simulink model "main_model"  (R2018b)
settings: Solver=VariableStepAuto  StartTime=0.0  StopTime=1  RelTol=1e-10
values from neighbouring files (symbols this model uses):
  ba = Jeq*omega_pos*n;       disp("    ba = " + ba)    [control_design.m]
  beq = bm + bl/r^2    (= 1.5e-05)    [data.m]
  Cts = 1.091    [data.m]
  Jeq = Jm + Jl/r^2    (= 5.65099476805e-06)    [data.m]
  ksa = Jeq*omega_pos^2*n;    disp("    ksa = " + ksa)    [control_design.m]
  ksia = Jeq*omega_pos^3;     disp("    ksia = " + ksia)    [control_design.m]
  lambda_rm = 0.01546    [data.m]
  Ld = 6.6e-3    (= 0.0066)    [data.m]
  Lls = 0.8e-3    (= 0.0008)    [data.m]
  Lq = 5.8e-3    (= 0.0058)    [data.m]
  Pp = 3    [data.m]
  r = 314.3008    [data.m]
  R0p = Lls*p;    disp("    R0p = " + R0p)    [control_design.m]    (also in torque_modulator.m = Lls*p;    disp("R0p = " + R0p))
  Rdp = Ld*p;     disp("    Rdp = " + Rdp)    [control_design.m]    (also in torque_modulator.m = Ld*p;     disp("Rdp = " + Rdp))
  Rqp = Lq*p;     disp("    Rqp = " + Rqp)    [control_design.m]    (also in torque_modulator.m = Lq*p;     disp("Rqp = " + Rqp))
  Rs = 1.02    [data.m]
  Rts_amb = 55    [data.m]
  Tamb_max = 40    [data.m]
undefined symbols (not defined in the file or in its folder): lamb
settings Model: Creator=Acer  LastModifiedBy=Acer

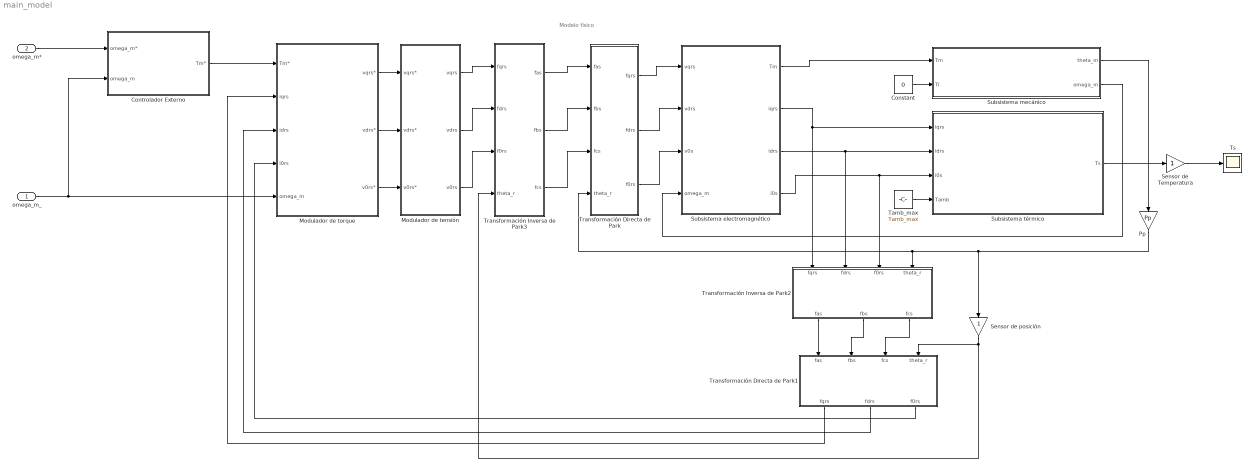
== system main_model ==
  note: Modelo físico
  omega_m_ : Inport
  omega_m* : Inport  Port=2
  " Sensor de posición" : Gain
  Constant : Constant  Value=0
  Controlador Externo : Subsystem
  Modulador de tensión : Subsystem
  Modulador de torque : Subsystem
  Pp : Gain  Gain=Pp
  Sensor de Temperatura : Gain
  Subsistema electromagnético : Subsystem
  Subsistema mecánico : Subsystem
  Subsistema térmico : Subsystem
  Tamb_max : Constant  Value=Tamb_max
  Transformación Directa de Park : MATLAB Function  TreatAsAtomicUnit=on
  Transformación Directa de Park1 : MATLAB Function  TreatAsAtomicUnit=on
  Transformación Inversa de Park2 : MATLAB Function  TreatAsAtomicUnit=on
  Transformación Inversa de Park3 : MATLAB Function  TreatAsAtomicUnit=on
  Ts : Scope
  wires:
  Subsistema mecánico/1(theta_m) -> Pp/1
  Subsistema mecánico/2(omega_m) -> Subsistema electromagnético/4(omega_m)
  Subsistema electromagnético/2(iqrs) -> Transformación Inversa de Park2/1(fqrs), Subsistema térmico/1(iqrs)
  Subsistema electromagnético/1(Tm) -> Subsistema mecánico/1(Tm)
  Subsistema electromagnético/4(i0s) -> Subsistema térmico/3(i0s), Transformación Inversa de Park2/3(f0rs)
  Subsistema térmico/1(Ts) -> Sensor de Temperatura/1
  Tamb_max/1 -> Subsistema térmico/4(Tamb)
  Pp/1 -> " Sensor de posición"/1, Transformación Directa de Park/4(theta_r), Transformación Inversa de Park2/4(theta_r)
  Subsistema electromagnético/3(idrs) -> Subsistema térmico/2(idrs), Transformación Inversa de Park2/2(fdrs)
  Modulador de tensión/1(vqrs) -> Transformación Inversa de Park3/1(fqrs)
  Modulador de tensión/2(vdrs) -> Transformación Inversa de Park3/2(fdrs)
  Modulador de tensión/3(v0rs) -> Transformación Inversa de Park3/3(f0rs)
  Controlador Externo/1(Tm*) -> Modulador de torque/1(Tm*)
  Transformación Directa de Park1/3(f0rs) -> Modulador de torque/4(i0rs)
  Modulador de torque/1(vqrs*) -> Modulador de tensión/1(vqrs*)
  Modulador de torque/2(vdrs*) -> Modulador de tensión/2(vdrs*)
  Modulador de torque/3(v0rs*) -> Modulador de tensión/3(v0rs*)
  Transformación Inversa de Park3/1(fas) -> Transformación Directa de Park/1(fas)
  Transformación Inversa de Park3/2(fbs) -> Transformación Directa de Park/2(fbs)
  Transformación Inversa de Park3/3(fcs) -> Transformación Directa de Park/3(fcs)
  Transformación Directa de Park/1(fqrs) -> Subsistema electromagnético/1(vqrs)
  Transformación Directa de Park/2(fdrs) -> Subsistema electromagnético/2(vdrs)
  Transformación Directa de Park/3(f0rs) -> Subsistema electromagnético/3(v0s)
  Constant/1 -> Subsistema mecánico/2(Tl)
  " Sensor de posición"/1 -> Transformación Inversa de Park3/4(theta_r), Transformación Directa de Park1/4(theta_r)
  Transformación Inversa de Park2/3(fcs) -> Transformación Directa de Park1/3(fcs)
  Transformación Inversa de Park2/2(fbs) -> Transformación Directa de Park1/2(fbs)
  Transformación Inversa de Park2/1(fas) -> Transformación Directa de Park1/1(fas)
  Transformación Directa de Park1/2(fdrs) -> Modulador de torque/3(idrs)
  Transformación Directa de Park1/1(fqrs) -> Modulador de torque/2(iqrs)
  Sensor de Temperatura/1 -> Ts/1
  omega_m*/1 -> Controlador Externo/1(omega_m*)
  omega_m_/1 -> Controlador Externo/2(omega_m), Modulador de torque/5(omega_m)

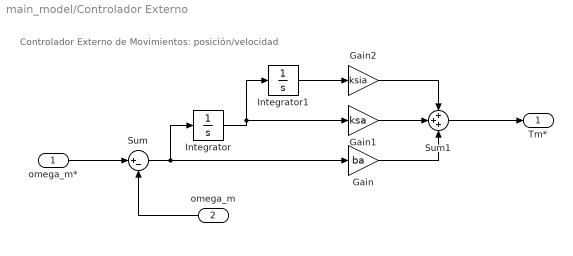
== system main_model/Controlador Externo ==
  note: Controlador Externo de Movimientos: posición/velocidad
  omega_m* : Inport
  omega_m : Inport  Port=2
  Gain : Gain  Gain=ba
  Gain1 : Gain  Gain=ksa
  Gain2 : Gain  Gain=ksia
  Integrator : Integrator
  Integrator1 : Integrator
  Sum : Sum  Inputs=|+-
  Sum1 : Sum  Inputs=+++
  Tm* : Outport
  wires:
  Integrator/1 -> Integrator1/1, Gain1/1
  Sum/1 -> Gain/1, Integrator/1
  Gain1/1 -> Sum1/2
  Gain/1 -> Sum1/3
  Integrator1/1 -> Gain2/1
  Gain2/1 -> Sum1/1
  omega_m/1 -> Sum/2
  Sum1/1 -> Tm*/1
  omega_m*/1 -> Sum/1

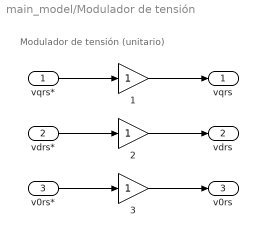
== system main_model/Modulador de tensión ==
  note: Modulador de tensión (unitario)
  vqrs* : Inport
  vdrs* : Inport  Port=2
  v0rs* : Inport  Port=3
  1 : Gain
  2 : Gain
  3 : Gain
  vqrs : Outport
  vdrs : Outport  Port=2
  v0rs : Outport  Port=3
  wires:
  vqrs*/1 -> 1/1
  vdrs*/1 -> 2/1
  1/1 -> vqrs/1
  v0rs*/1 -> 3/1
  2/1 -> vdrs/1
  3/1 -> v0rs/1

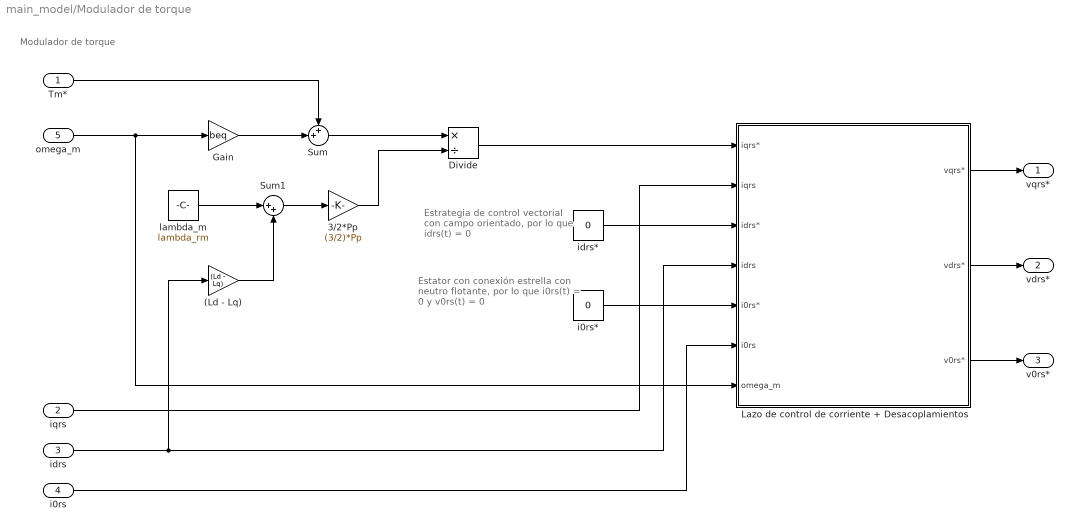
== system main_model/Modulador de torque ==
  note: Modulador de torque
  note: Estator con conexión estrella
      | con neutro flotante,
      | por lo que i0rs(t) = 0 y v0rs(t) = 0
  note: Estrategia de control vectorial
      | con campo orientado,
      | por lo que idrs(t) = 0
  Tm* : Inport
  iqrs : Inport  Port=2
  idrs : Inport  Port=3
  i0rs : Inport  Port=4
  omega_m : Inport  Port=5
  (Ld - Lq) : Gain  Gain=(Ld - Lq)
  3/2*Pp : Gain  Gain=(3/2)*Pp
  Divide : Product  Inputs=*/
  Gain : Gain  Gain=beq
  Lazo de control de corriente + Desacoplamientos : Subsystem
  Sum : Sum  Inputs=++|
  Sum1 : Sum  Inputs=|++
  i0rs* : Constant  Value=0
  idrs* : Constant  Value=0
  lambda_m : Constant  Value=lambda_rm
  vqrs* : Outport
  vdrs* : Outport  Port=2
  v0rs* : Outport  Port=3
  wires:
  omega_m/1 -> Gain/1, Lazo de control de corriente + Desacoplamientos/7(omega_m)
  i0rs*/1 -> Lazo de control de corriente + Desacoplamientos/5(i0rs*)
  3/2*Pp/1 -> Divide/2
  (Ld - Lq)/1 -> Sum1/2
  Sum1/1 -> 3/2*Pp/1
  Divide/1 -> Lazo de control de corriente + Desacoplamientos/1(iqrs*)
  Gain/1 -> Sum/2
  idrs*/1 -> Lazo de control de corriente + Desacoplamientos/3(idrs*)
  Sum/1 -> Divide/1
  idrs/1 -> (Ld - Lq)/1, Lazo de control de corriente + Desacoplamientos/4(idrs)
  i0rs/1 -> Lazo de control de corriente + Desacoplamientos/6(i0rs)
  iqrs/1 -> Lazo de control de corriente + Desacoplamientos/2(iqrs)
  lambda_m/1 -> Sum1/1
  Tm*/1 -> Sum/1
  Lazo de control de corriente + Desacoplamientos/1(vqrs*) -> vqrs*/1
  Lazo de control de corriente + Desacoplamientos/3(v0rs*) -> v0rs*/1
  Lazo de control de corriente + Desacoplamientos/2(vdrs*) -> vdrs*/1

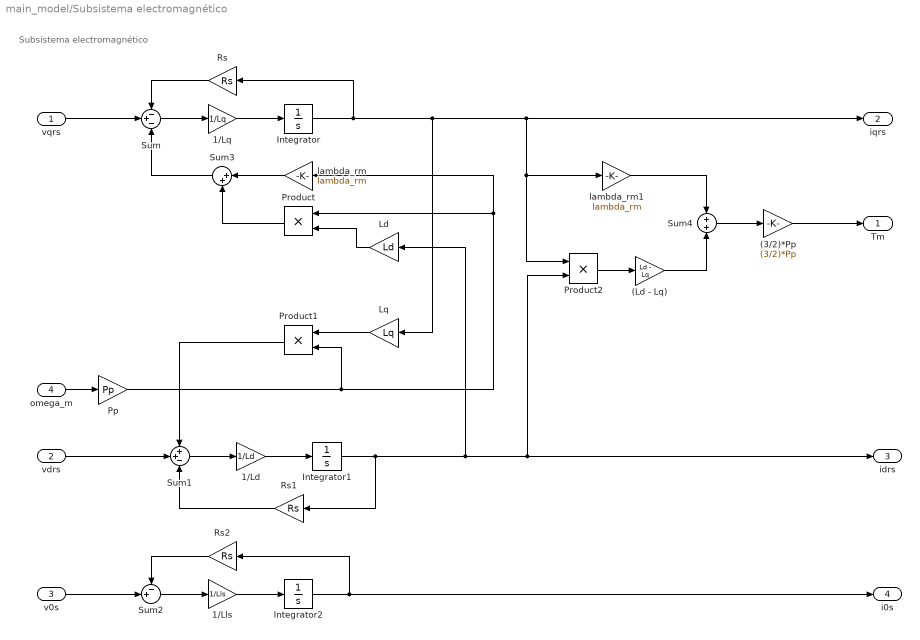
== system main_model/Subsistema electromagnético ==
  note: Subsistema electromagnético
  vqrs : Inport
  vdrs : Inport  Port=2
  v0s : Inport  Port=3
  omega_m : Inport  Port=4
  (3/2)*Pp : Gain  Gain=(3/2)*Pp
  (Ld - Lq) : Gain  Gain=Ld - Lq
  1/Ld : Gain  Gain=1/Ld
  1/Lls : Gain  Gain=1/Lls
  1/Lq : Gain  Gain=1/Lq
  Integrator : Integrator
  Integrator1 : Integrator
  Integrator2 : Integrator
  Ld : Gain  Gain=Ld
  Lq : Gain  Gain=Lq
  Pp : Gain  Gain=Pp
  Product : Product
  Product1 : Product
  Product2 : Product
  Rs : Gain  Gain=Rs
  Rs1 : Gain  Gain=Rs
  Rs2 : Gain  Gain=Rs
  Sum : Sum  Inputs=-+-
  Sum1 : Sum  Inputs=++-
  Sum2 : Sum  Inputs=-+|
  Sum3 : Sum  Inputs=|++
  Sum4 : Sum  Inputs=+|+
  lambda_rm : Gain  Gain=lambda_rm
  lambda_rm1 : Gain  Gain=lambda_rm
  Tm : Outport
  iqrs : Outport  Port=2
  idrs : Outport  Port=3
  i0s : Outport  Port=4
  wires:
  lambda_rm/1 -> Sum3/1
  Product1/1 -> Sum1/1
  Lq/1 -> Product1/1
  Pp/1 -> lambda_rm/1, Product/1, Product1/2
  Product/1 -> Sum3/2
  vdrs/1 -> Sum1/2
  1/Lq/1 -> Integrator/1
  vqrs/1 -> Sum/2
  omega_m/1 -> Pp/1
  Integrator1/1 -> Ld/1, Product2/2, idrs/1, Rs1/1
  Sum1/1 -> 1/Ld/1
  Integrator/1 -> Rs/1, Lq/1, iqrs/1, Product2/1, lambda_rm1/1
  Sum2/1 -> 1/Lls/1
  Integrator2/1 -> i0s/1, Rs2/1
  Sum3/1 -> Sum/3
  Rs1/1 -> Sum1/3
  Sum4/1 -> (3/2)*Pp/1
  Ld/1 -> Product/2
  lambda_rm1/1 -> Sum4/1
  (3/2)*Pp/1 -> Tm/1
  1/Ld/1 -> Integrator1/1
  Rs2/1 -> Sum2/1
  Rs/1 -> Sum/1
  Product2/1 -> (Ld - Lq)/1
  (Ld - Lq)/1 -> Sum4/2
  Sum/1 -> 1/Lq/1
  1/Lls/1 -> Integrator2/1
  v0s/1 -> Sum2/2

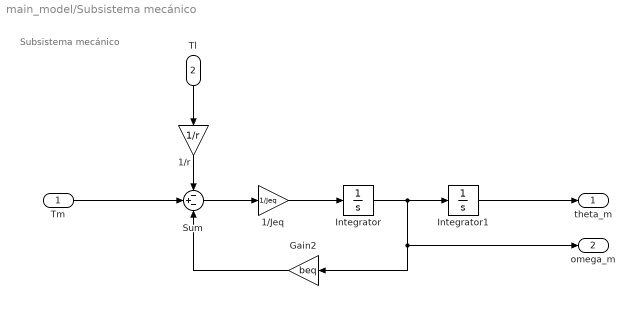
== system main_model/Subsistema mecánico ==
  note: Subsistema mecánico
  Tm : Inport
  Tl : Inport  Port=2
  1/Jeq : Gain  Gain=1/Jeq
  1/r : Gain  Gain=1/r
  Gain2 : Gain  Gain=beq
  Integrator : Integrator
  Integrator1 : Integrator
  Sum : Sum  Inputs=-+-
  theta_m : Outport
  omega_m : Outport  Port=2
  wires:
  Integrator1/1 -> theta_m/1
  Integrator/1 -> omega_m/1, Gain2/1, Integrator1/1
  Tm/1 -> Sum/2
  1/r/1 -> Sum/1
  Sum/1 -> 1/Jeq/1
  Tl/1 -> 1/r/1
  Gain2/1 -> Sum/3
  1/Jeq/1 -> Integrator/1

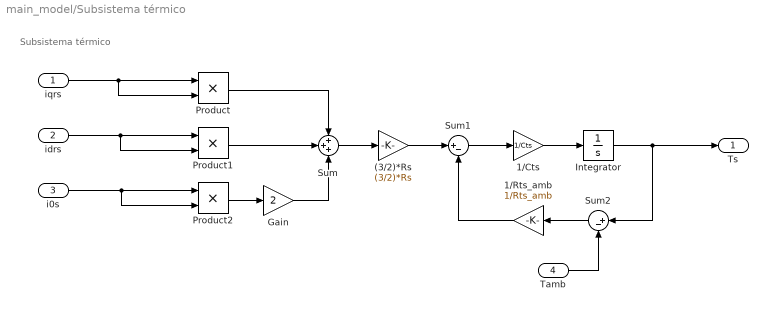
== system main_model/Subsistema térmico ==
  note: Subsistema térmico
  iqrs : Inport
  idrs : Inport  Port=2
  i0s : Inport  Port=3
  Tamb : Inport  Port=4
  (3/2)*Rs : Gain  Gain=(3/2)*Rs
  1/Cts : Gain  Gain=1/Cts
  1/Rts_amb : Gain  Gain=1/Rts_amb
  Gain : Gain  Gain=2
  Integrator : Integrator  InitialCondition=Tamb_max
  Product : Product
  Product1 : Product
  Product2 : Product
  Sum : Sum  Inputs=+++
  Sum1 : Sum  Inputs=|+-
  Sum2 : Sum  Inputs=|+-
  Ts : Outport
  wires:
  Integrator/1 -> Ts/1, Sum2/1
  1/Cts/1 -> Integrator/1
  i0s/1 -> Product2/2, Product2/1
  Product/1 -> Sum/1
  Sum2/1 -> 1/Rts_amb/1
  (3/2)*Rs/1 -> Sum1/1
  Tamb/1 -> Sum2/2
  Sum/1 -> (3/2)*Rs/1
  1/Rts_amb/1 -> Sum1/2
  Gain/1 -> Sum/3
  Sum1/1 -> 1/Cts/1
  iqrs/1 -> Product/2, Product/1
  idrs/1 -> Product1/2, Product1/1
  Product2/1 -> Gain/1
  Product1/1 -> Sum/2

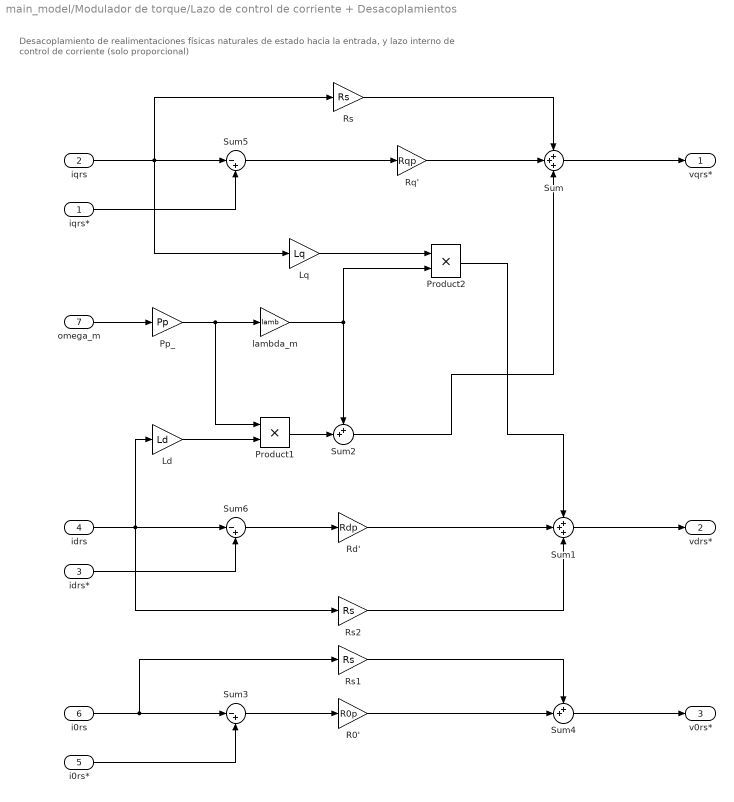
== system main_model/Modulador de torque/Lazo de control de corriente + Desacoplamientos ==
  note: Desacoplamiento de realimentaciones físicas naturales de estado hacia la entrada,
      | y lazo interno de control de corriente (solo proporcional)
  iqrs* : Inport
  iqrs : Inport  Port=2
  idrs* : Inport  Port=3
  idrs : Inport  Port=4
  i0rs* : Inport  Port=5
  i0rs : Inport  Port=6
  omega_m : Inport  Port=7
  Ld : Gain  Gain=Ld
  Lq : Gain  Gain=Lq
  Pp_ : Gain  Gain=Pp
  Product1 : Product
  Product2 : Product
  R0' : Gain  Gain=R0p
  Rd' : Gain  Gain=Rdp
  Rq' : Gain  Gain=Rqp
  Rs : Gain  Gain=Rs
  Rs1 : Gain  Gain=Rs
  Rs2 : Gain  Gain=Rs
  Sum : Sum  Inputs=+++
  Sum1 : Sum  Inputs=+++
  Sum2 : Sum  Inputs=++|
  Sum3 : Sum  Inputs=|-+
  Sum4 : Sum  Inputs=++|
  Sum5 : Sum  Inputs=|-+
  Sum6 : Sum  Inputs=|-+
  lambda_m : Gain  Gain=lamb
  vqrs* : Outport
  vdrs* : Outport  Port=2
  v0rs* : Outport  Port=3
  wires:
  omega_m/1 -> Pp_/1
  lambda_m/1 -> Product2/2, Sum2/1
  i0rs*/1 -> Sum3/2
  Pp_/1 -> Product1/1, lambda_m/1
  Rq'/1 -> Sum/2
  R0'/1 -> Sum4/2
  i0rs/1 -> Sum3/1, Rs1/1
  Sum3/1 -> R0'/1
  Sum4/1 -> v0rs*/1
  Sum1/1 -> vdrs*/1
  Product2/1 -> Sum1/1
  idrs*/1 -> Sum6/2
  Sum/1 -> vqrs*/1
  Sum6/1 -> Rd'/1
  idrs/1 -> Ld/1, Rs2/1, Sum6/1
  Sum5/1 -> Rq'/1
  iqrs/1 -> Lq/1, Sum5/1, Rs/1
  Lq/1 -> Product2/1
  Sum2/1 -> Sum/3
  Rs2/1 -> Sum1/3
  Rs1/1 -> Sum4/1
  Rs/1 -> Sum/1
  Rd'/1 -> Sum1/2
  Ld/1 -> Product1/2
  iqrs*/1 -> Sum5/2
  Product1/1 -> Sum2/2

== matlab function main_model/Transformación Inversa de Park2 ==
  data: fqrs input; fdrs input; f0rs input; theta_r input; fas output; fbs output; fcs output
function [fas, fbs, fcs] = dq0_inverse( fqrs, fdrs, f0rs, theta_r )
% TRANSFORMACIÓN INVERSA DE PARK
%   Transformación directa para pasar desde coordenadas trifásicas del
%   estator abc a las coordenadas fijas al rotor qd0.
fqd0 = [ fqrs; fdrs; f0rs ];

A = [ 
    cos(theta_r)            sin(theta_r)            1;
    cos(theta_r - 2*pi/3)   sin(theta_r - 2*pi/3)   1;
    cos(theta_r + 2*pi/3)   sin(theta_r + 2*pi/3)   1
    ];

fabc =  A * fqd0;

fas = fabc(1);
fbs = fabc(2);
fcs = fabc(3);

end

== matlab function main_model/Transformación Directa de Park ==
  data: fas input; fbs input; fcs input; theta_r input; fqrs output; fdrs output; f0rs output
function [fqrs, fdrs, f0rs] = dq0_direct( fas, fbs, fcs, theta_r )
% TRANSFORMACIÓN DIRECTA DE PARK
%   Transformación directa para pasar desde coordenadas trifásicas del
%   estator abc a las coordenadas fijas al rotor qd0.
fabc = [ fas; fbs; fcs ];

A = [ 
    cos(theta_r)    cos(theta_r - 2*pi/3)   cos(theta_r + 2*pi/3);
    sin(theta_r)    sin(theta_r - 2*pi/3)   sin(theta_r + 2*pi/3);
    0.5             0.5                     0.5
    ];

fqd0 = (2/3) * A * fabc;

fqrs = fqd0(1);
fdrs = fqd0(2);
f0rs = fqd0(3);

end

== matlab function main_model/Transformación Directa de Park1 ==
  data: fas input; fbs input; fcs input; theta_r input; fqrs output; fdrs output; f0rs output
function [fqrs, fdrs, f0rs] = dq0_direct( fas, fbs, fcs, theta_r )
% TRANSFORMACIÓN DIRECTA DE PARK
%   Transformación directa para pasar desde coordenadas trifásicas del
%   estator abc a las coordenadas fijas al rotor qd0.
fabc = [ fas; fbs; fcs ];

A = [ 
    cos(theta_r)    cos(theta_r - 2*pi/3)   cos(theta_r + 2*pi/3);
    sin(theta_r)    sin(theta_r - 2*pi/3)   sin(theta_r + 2*pi/3);
    0.5             0.5                     0.5
    ];

fqd0 = (2/3) * A * fabc;

fqrs = fqd0(1);
fdrs = fqd0(2);
f0rs = fqd0(3);

end

== matlab function main_model/Transformación Inversa de Park3 ==
  data: fqrs input; fdrs input; f0rs input; theta_r input; fas output; fbs output; fcs output
function [fas, fbs, fcs] = dq0_inverse( fqrs, fdrs, f0rs, theta_r )
% TRANSFORMACIÓN INVERSA DE PARK
%   Transformación directa para pasar desde coordenadas trifásicas del
%   estator abc a las coordenadas fijas al rotor qd0.
fqd0 = [ fqrs; fdrs; f0rs ];

A = [ 
    cos(theta_r)            sin(theta_r)            1;
    cos(theta_r - 2*pi/3)   sin(theta_r - 2*pi/3)   1;
    cos(theta_r + 2*pi/3)   sin(theta_r + 2*pi/3)   1
    ];

fabc =  A * fqd0;

fas = fabc(1);
fbs = fabc(2);
fcs = fabc(3);

end
